simulink model "tuning_motorFBD"  (R2022a)
settings: Solver=VariableStepAuto  StartTime=0.0  StopTime=10.0  RelTol=1e-3
values from neighbouring files (symbols this model uses):
  g = 9.81    [LQRCalcs.m]    (also in cf_firstOrderStateMdl.m; init_parameters.m; main.m; parameters_buildingSimulink.m)
  Gamma = [cT, cT, cT, cT ... (first row only)    [init_parameters.m]    (also in parameters_buildingSimulink.m; parameters_init.m; parameters_init2.m; parameters_init____CodeToImplementLater.m)
  GammaInv = inv(Gamma)    [init_parameters.m]    (also in parameters_buildingSimulink.m; parameters_init.m; parameters_init2.m)
  J = cat(2, [0 0 0]', J)    [LQRCalcs.m]    (also in init_parameters.m = diag([0.082, 0.0845, 0.1377]); main.m = diag([0.082, 0.0845, 0.1377]); parameters_buildingSimulink.m = diag([0.082, 0.0845, 0.1377]); parameters_init.m = diag([0.082, 0.0845, 0.1377]))
  J_inv = inv(J)    [main.m]    (also in parameters_init.m; parameters_init2.m)
  m = 0.003    [LQRCalcs.m]    (also in cf_firstOrderStateMdl.m; init_parameters.m = 4.34; main.m = 4.34; parameters_buildingSimulink.m = 4.34)
undefined symbols (not defined in the file or in its folder): Gain
libraries: matrix_library x1, aerolibutil x1, sharedtransform x1
settings Model: Creator=willg  LastModifiedBy=willg

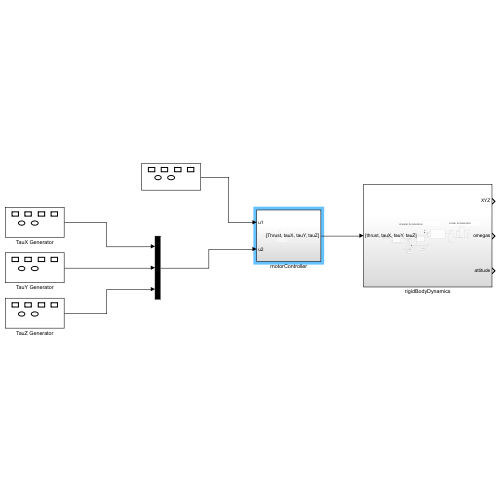
[thumbnail: Simulink's stored preview of the top-level diagram]
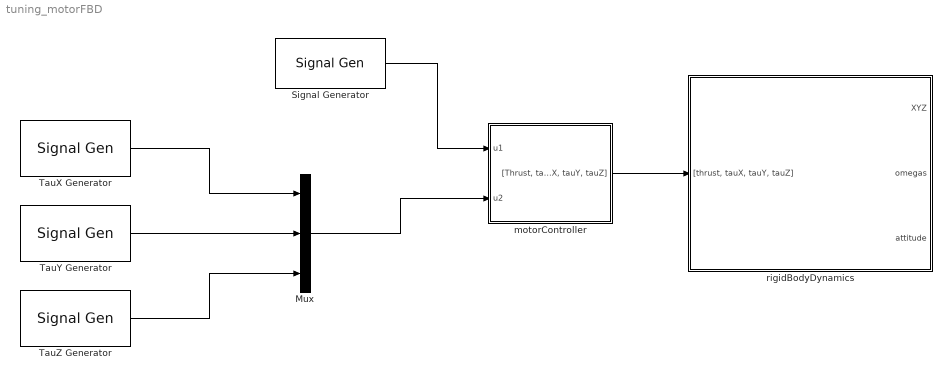
== system tuning_motorFBD ==
  Mux : Mux  Inputs=3
  Signal Generator : SignalGenerator  Amplitude=2*m*g
  TauX Generator : SignalGenerator  Amplitude=0  Frequency=50
  TauY Generator : SignalGenerator  Amplitude=0  Frequency=50
  TauZ Generator : SignalGenerator  Amplitude=0  Frequency=50
  motorController : Subsystem
  rigidBodyDynamics : Subsystem
  wires:
  motorController/1("[Thrust, tauX, tauY, tauZ]") -> rigidBodyDynamics/1("[thrust, tauX, tauY, tauZ]")
  Mux/1 -> motorController/2(u2)
  Signal Generator/1 -> motorController/1(u1)
  TauY Generator/1 -> Mux/2
  TauX Generator/1 -> Mux/1
  TauZ Generator/1 -> Mux/3

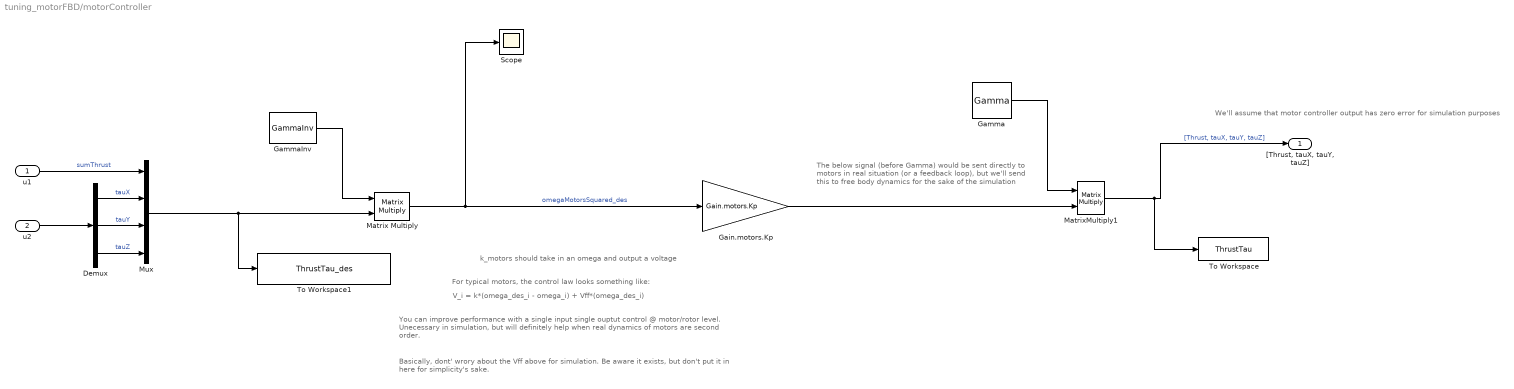
== system tuning_motorFBD/motorController ==
  note: We'll assume that motor controller output has zero error for simulation purposes
  note: The below signal (before Gamma) would be sent directly to motors in real situation (or a feedback loop), but we'll send this to free body dynamics for the sake of the simulation
  note: k_motors should take in an omega and output a voltage
  note: Basically, dont' wrory about the Vff above for simulation. Be aware it exists, but don't put it in here for simplicity's sake.
  note: You can improve performance with a single input single ouptut control @ motor/rotor level. Unecessary in simulation, but will definitely help when real dynamics of motors are second order.
  note: V_i = k*(omega_des_i - omega_i) + Vff*(omega_des_i)
  note: For typical motors, the control law looks something like:
  u1 : Inport
  u2 : Inport  Port=2
  Demux : Demux  Outputs=3
  Gain.motors.Kp : Gain  Gain=Gain.motors.Kp
  Gamma : Constant  Value=Gamma
  GammaInv : Constant  Value=GammaInv
  Matrix Multiply : Product  Multiplication=Matrix(*)
  MatrixMultiply1 : Product  Multiplication=Matrix(*)
  Mux : Mux
  Scope : Scope
  To Workspace : ToWorkspace  VariableName=ThrustTau  SaveFormat=Timeseries  SampleTime=-1
  To Workspace1 : ToWorkspace  VariableName=ThrustTau_des  SaveFormat=Timeseries  SampleTime=-1
  "[Thrust, tauX, tauY, tauZ]" : Outport
  wires:
  u2/1 -> Demux/1
  u1/1 -> Mux/1  "sumThrust"
  Demux/2 -> Mux/3  "tauY"
  Demux/1 -> Mux/2  "tauX"
  Demux/3 -> Mux/4  "tauZ"
  Gamma/1 -> MatrixMultiply1/1
  MatrixMultiply1/1 -> To Workspace/1, "[Thrust, tauX, tauY, tauZ]"/1  "[Thrust, tauX, tauY, tauZ]"
  Mux/1 -> To Workspace1/1, Matrix Multiply/2
  GammaInv/1 -> Matrix Multiply/1
  Matrix Multiply/1 -> Scope/1, Gain.motors.Kp/1  "omegaMotorsSquared_des"
  Gain.motors.Kp/1 -> MatrixMultiply1/2

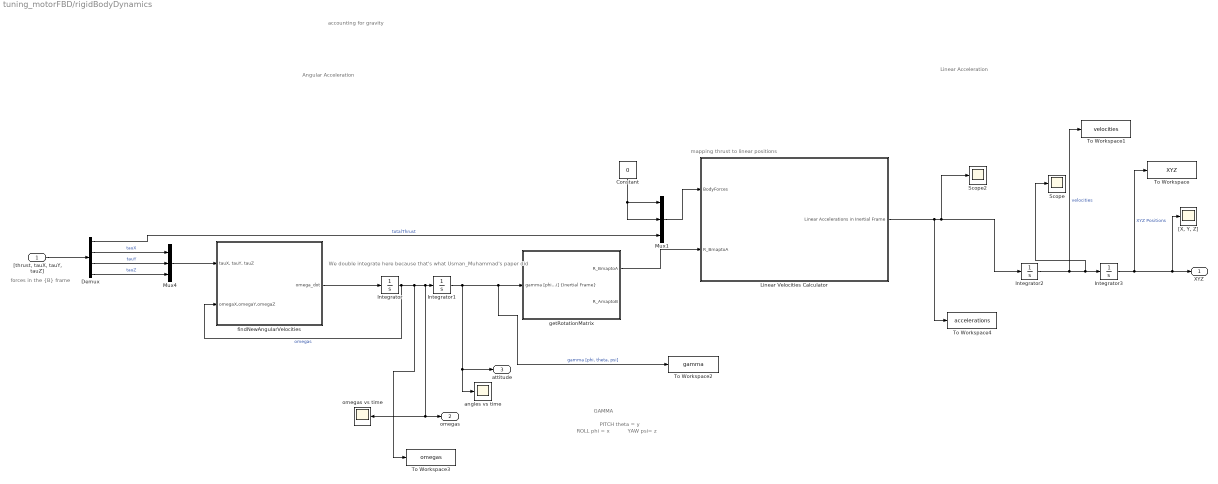
== system tuning_motorFBD/rigidBodyDynamics ==
  note: mapping thrust to linear positions
  note: We double integrate here because that's what Usman_Muhammad's paper did
  note: Angular Acceleration
  note: Linear Acceleration
  note: GAMMA
  note: accounting for gravity
  note: forces in the {B} frame
  note: ROLL
      | phi = x
  note: PITCH
      | theta = y
  note: YAW
      | psi= z
  "[thrust, tauX, tauY, tauZ]" : Inport
  Constant : Constant  Value=0
  Demux : Demux
  Integrator{,1..3} (4 alike) : Integrator
  Linear Velocities Calculator : Subsystem
  Mux1 : Mux  Inputs=3
  Mux4 : Mux  Inputs=3
  Scope : Scope
  Scope2 : Scope
  To Workspace : ToWorkspace  VariableName=XYZ  SaveFormat=Timeseries  SampleTime=-1
  To Workspace1 : ToWorkspace  VariableName=velocities  SaveFormat=Timeseries  SampleTime=-1
  To Workspace2 : ToWorkspace  VariableName=gamma  SaveFormat=Timeseries  SampleTime=-1
  To Workspace3 : ToWorkspace  VariableName=omegas  SaveFormat=Timeseries  SampleTime=-1
  To Workspace4 : ToWorkspace  VariableName=accelerations  SaveFormat=Timeseries  SampleTime=-1
  "[X, Y, Z]" : Scope
  angles vs time : Scope
  findNewAngularVelocities : Subsystem
  getRotationMatrix : Subsystem
  omegas vs time : Scope
  XYZ : Outport
  omegas : Outport  Port=2
  attitude : Outport  Port=3
  wires:
  Demux/2 -> Mux4/1  "tauX"
  Demux/4 -> Mux4/3  "tauZ"
  Demux/3 -> Mux4/2  "tauY"
  Constant/1 -> Mux1/2, Mux1/1
  Demux/1 -> Mux1/3  "totalThrust"
  "[thrust, tauX, tauY, tauZ]"/1 -> Demux/1
  Integrator1/1 -> To Workspace2/1, getRotationMatrix/1("gamma [phi, theta, psi] {Inertial Frame}"), attitude/1, angles vs time/1  "gamma [phi, theta, psi]"
  findNewAngularVelocities/1(omega_dot) -> Integrator/1
  Integrator/1 -> To Workspace3/1, omegas vs time/1, omegas/1, Integrator1/1, findNewAngularVelocities/2(omegaX,omegaY,omegaZ)  "omegas"
  Mux4/1 -> findNewAngularVelocities/1("tauX, tauY, tauZ")
  Linear Velocities Calculator/1(Linear Accelerations in Inertial Frame) -> Integrator2/1, Scope2/1, To Workspace4/1
  Integrator2/1 -> To Workspace1/1, Integrator3/1, Scope/1  "velocities"
  Integrator3/1 -> "[X, Y, Z]"/1, XYZ/1, To Workspace/1  "XYZ Positions"
  Mux1/1 -> Linear Velocities Calculator/1(BodyForces)
  getRotationMatrix/1(R_BmaptoA) -> Linear Velocities Calculator/2(R_BmaptoA)

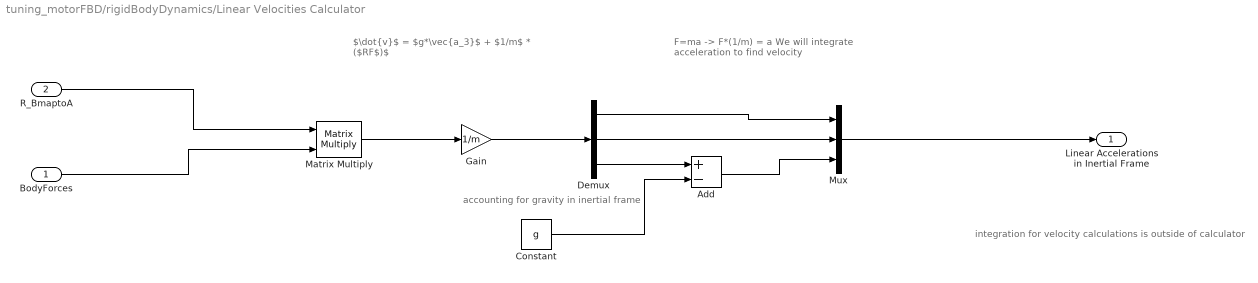
== system tuning_motorFBD/rigidBodyDynamics/Linear Velocities Calculator ==
  note: integration for velocity calculations is outside of calculator
  note: F=ma -> F*(1/m) = a
      | We will integrate acceleration to find velocity
  note: accounting for gravity in inertial frame
  note: $\dot{v}$ = $g*\vec{a_3}$ + $1/m$ * ($RF$)$
  BodyForces : Inport
  R_BmaptoA : Inport  Port=2
  Add : Sum  Inputs=+-
  Constant : Constant  Value=g
  Demux : Demux  Outputs=3
  Gain : Gain  Gain=1/m
  Matrix Multiply : Product  Multiplication=Matrix(*)
  Mux : Mux  Inputs=3
  Linear Accelerations in Inertial Frame : Outport
  wires:
  BodyForces/1 -> Matrix Multiply/2
  R_BmaptoA/1 -> Matrix Multiply/1
  Matrix Multiply/1 -> Gain/1
  Gain/1 -> Demux/1
  Demux/3 -> Add/1
  Constant/1 -> Add/2
  Add/1 -> Mux/3
  Demux/2 -> Mux/2
  Demux/1 -> Mux/1
  Mux/1 -> Linear Accelerations in Inertial Frame/1

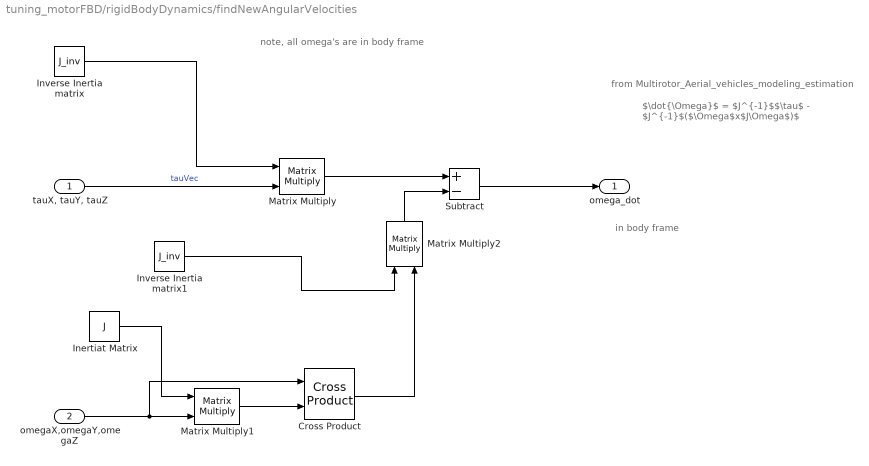
== system tuning_motorFBD/rigidBodyDynamics/findNewAngularVelocities ==
  note: from Multirotor_Aerial_vehicles_modeling_estimation
  note: note, all omega's are in body frame
  note: $\dot{\Omega}$ = $J^{-1}$$\tau$ - $J^{-1}$($\Omega$x$J\Omega$)$
  note: in body frame
  "tauX, tauY, tauZ" : Inport
  omegaX,omegaY,omegaZ : Inport  Port=2
  Cross Product : matrix_library/Cross Product
      settings: SourceProductBaseCode=SL
  Inertiat Matrix : Constant  Value=J
  Inverse Inertia matrix : Constant  Value=J_inv
  Inverse Inertia matrix1 : Constant  Value=J_inv
  Matrix Multiply : Product  Multiplication=Matrix(*)
  Matrix Multiply1 : Product  Multiplication=Matrix(*)
  Matrix Multiply2 : Product  Multiplication=Matrix(*)
  Subtract : Sum  Inputs=+-
  omega_dot : Outport
  wires:
  "tauX, tauY, tauZ"/1 -> Matrix Multiply/2  "tauVec"
  Matrix Multiply/1 -> Subtract/1
  Inverse Inertia matrix/1 -> Matrix Multiply/1
  Inertiat Matrix/1 -> Matrix Multiply1/1
  omegaX,omegaY,omegaZ/1 -> Cross Product/1, Matrix Multiply1/2
  Matrix Multiply1/1 -> Cross Product/2
  Inverse Inertia matrix1/1 -> Matrix Multiply2/1
  Cross Product/1 -> Matrix Multiply2/2
  Matrix Multiply2/1 -> Subtract/2
  Subtract/1 -> omega_dot/1

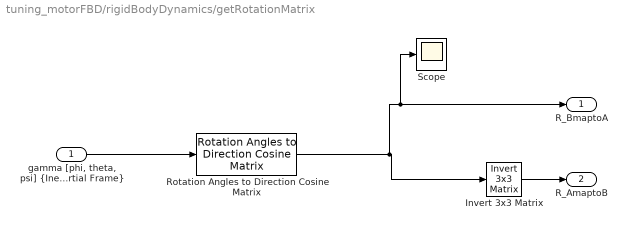
== system tuning_motorFBD/rigidBodyDynamics/getRotationMatrix ==
  "gamma [phi, theta, psi] {Inertial Frame}" : Inport
  Invert 3x3 Matrix : aerolibutil/Invert  3x3 Matrix
  Rotation Angles to Direction Cosine Matrix : sharedtransform/Rotation Angles to Direction Cosine Matrix  rotationOrder=ZYX  aMode=aMode
      settings: SourceProductBaseCode=AE,PW,DR,MT,VE
  Scope : Scope
  R_BmaptoA : Outport
  R_AmaptoB : Outport  Port=2
  wires:
  "gamma [phi, theta, psi] {Inertial Frame}"/1 -> Rotation Angles to Direction Cosine Matrix/1
  Rotation Angles to Direction Cosine Matrix/1 -> Scope/1, R_BmaptoA/1, Invert 3x3 Matrix/1
  Invert 3x3 Matrix/1 -> R_AmaptoB/1
